simulink model "esempio4S"  (R2021a)
settings: Solver=VariableStepAuto  StartTime=0.0  StopTime=10.0  RelTol=1e-3
values from neighbouring files (symbols this model uses):
  A = [0 1; 0 -2]    [esempio1.m]    (also in esempio2.m = [-1 -4; 1 -1]; esempio3.m = [-1 -2; 1 -1]; esempio4.m = [0 1; -25 0])
  Ao = A-L*C    [esempio1.m]    (also in esempio2.m; esempio3.m; esempio4.m)
  B = [0; 1]    [esempio1.m]    (also in esempio2.m = [0;1]; esempio3.m = [0;1]; esempio4.m = [0;1])
  Bo = [B L]    [esempio1.m]    (also in esempio2.m; esempio3.m; esempio4.m)
  C = [1 0]    [esempio1.m]    (also in esempio2.m; esempio3.m; esempio4.m = [0 1])
  Co = eye(2)    [esempio1.m]    (also in esempio2.m; esempio3.m; esempio4.m)
  D = 0    [esempio1.m]    (also in esempio2.m; esempio3.m; esempio4.m)
  Do = zeros(2,2)    [esempio1.m]    (also in esempio2.m; esempio3.m; esempio4.m)
  K = place(A,B, [-2 -10])    [esempio2.m]    (also in esempio3.m = place(A,B, [-5 -15]); esempio4.m = place(A,B, [-1 -10]))
settings Model: Creator=itama  LastModifiedBy=itama

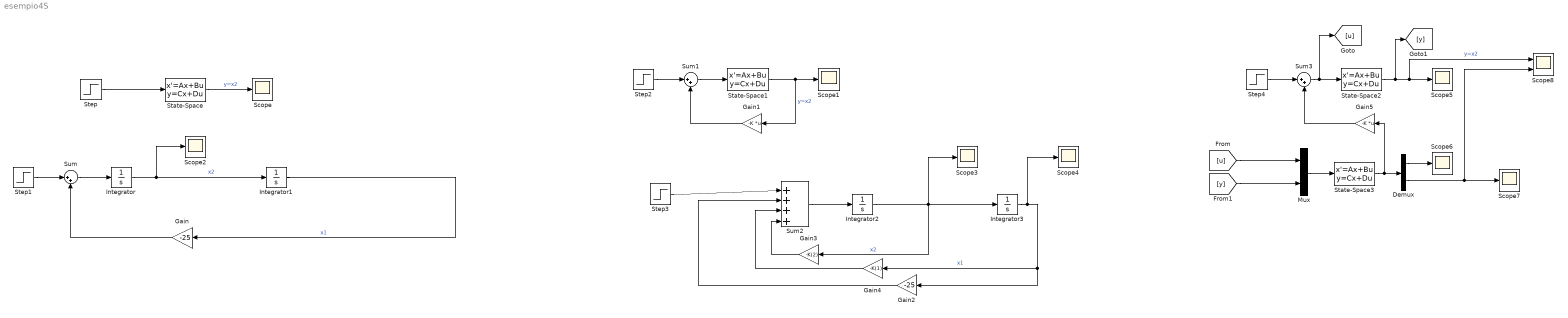
== system esempio4S ==
  Demux : Demux  Outputs=2
  Gain : Gain  Gain=-25
  Gain1 : Gain  Gain=-K  Multiplication=Matrix(K*u)
  Gain2 : Gain  Gain=-25
  Gain3 : Gain  Gain=-K(2)
  Gain4 : Gain  Gain=-K(1)
  Gain5 : Gain  Gain=-K  Multiplication=Matrix(K*u)
  Integrator{,1..3} (4 alike) : Integrator
  Mux : Mux  Inputs=2
  Scope{,1..7} (8 alike) : Scope
  Scope8 : Scope  NumInputPorts=2
  State-Space : StateSpace  A=A  B=B  C=C  D=D  InitialCondition=[0;0]
  State-Space1 : StateSpace  A=A  B=B  C=eye(2)  D=zeros(2,1)  InitialCondition=[0;0]
  State-Space2 : StateSpace  A=A  B=B  C=C  D=D  InitialCondition=[0;0]
  State-Space3 : StateSpace  A=Ao  B=Bo  C=Co  D=Do  InitialCondition=[0;0]
  Step : Step  Time=0  SampleTime=0
  Step1 : Step  SampleTime=0
  Step2 : Step  Time=0  SampleTime=0
  Step3 : Step  SampleTime=0
  Step4 : Step  Time=0  SampleTime=0
  Sum : Sum  Inputs=|++
  Sum1 : Sum  Inputs=|++
  Sum2 : Sum  Inputs=|++++
  Sum3 : Sum  Inputs=|++
  wires:
  Step/1 -> State-Space/1
  State-Space/1 -> Scope/1  "y=x2"
  Integrator/1 -> Scope2/1, Integrator1/1  "x2"
  Integrator1/1 -> Gain/1  "x1"
  Step1/1 -> Sum/1
  Gain/1 -> Sum/2
  Sum/1 -> Integrator/1
  State-Space1/1 -> Gain1/1, Scope1/1  "y=x2"
  Gain1/1 -> Sum1/2
  Step2/1 -> Sum1/1
  Sum1/1 -> State-Space1/1
  Step3/1 -> Sum2/1
  Integrator3/1 -> Scope4/1, Gain4/1, Gain2/1  "x1"
  Gain2/1 -> Sum2/2
  Integrator2/1 -> Gain3/1, Integrator3/1, Scope3/1  "x2"
  Gain3/1 -> Sum2/4
  Gain4/1 -> Sum2/3
  Sum2/1 -> Integrator2/1
  Sum3/1 -> [u], State-Space2/1
  State-Space2/1 -> [y], Scope8/1, Scope5/1  "y=x2"
  Step4/1 -> Sum3/1
  [u] -> Mux/1
  [y] -> Mux/2
  Mux/1 -> State-Space3/1
  State-Space3/1 -> Demux/1, Gain5/1
  Gain5/1 -> Sum3/2
  Demux/1 -> Scope6/1
  Demux/2 -> Scope8/2, Scope7/1
